simulink model "parrot_communication_host"  (R2022a)
settings: Solver=FixedStepAuto  StartTime=0.0  StopTime=50  FixedStep=0.05  RelTol=1e-3
undefined symbols (not defined in the file or in its folder): f
libraries: instrumentlib x2
settings Model: ExtModeTrigDuration=80  Creator=The MathWorks, Inc.  LastModifiedBy=The MathWorks, Inc.
settings SolverCC: AlgebraicLoopSolver=TrustRegion
settings DataIOCC: ReturnWorkspaceOutputs=off
settings OptimizationCC: DefaultParameterBehavior=Inlined  EnhancedBackFolding=on  PassReuseOutputArgsAs=Individual arguments  MaxStackSize=64  OptimizeBlockOrder=speed  DifferentSizesBufferReuse=on  OptimizationCustomize=off  EfficientTunableParamExpr=on
settings DebuggingCC: ParameterTunabilityLossMsg=error  UnconnectedInputMsg=warning  UnconnectedOutputMsg=warning  UnconnectedLineMsg=warning  SFMachineParentedDataDiag=warning  ArithmeticOperatorsInVariantConditions=warning
settings HardwareCC: ProdBitPerPointer=32  ProdBitPerSizeT=32  ProdBitPerPtrDiffT=32  ProdLargestAtomicInteger=Long  ProdWordSize=32  ProdHWDeviceType=ARM Compatible->ARM 9  UseEmbeddedCoderFeatures=off  UseSimulinkCoderFeatures=off
settings SFSimCC: SimUseLocalCustomCode=off  MATLABDynamicMemAlloc=off  CustomCodeUndefinedFunction=UseInterfaceOnly
settings RTWCC: SystemTargetFile=ert.tlc  TemplateMakefile=ert_default_tmf  GenerateReport=on  RTWUseLocalCustomCode=off  Toolchain=Sourcery G++ Lite GNU Toolchain for Drones  IncludeHyperlinkInReport=on  LaunchReport=on  GenerateTraceInfo=on  GenerateTraceReport=on  GenerateTraceReportSl=on  GenerateTraceReportSf=on  GenerateTraceReportEml=on
settings CodeAppCC: ForceParamTrailComments=on  IgnoreCustomStorageClasses=off  OperatorAnnotations=on  SimulinkDataObjDesc=on  SFDataObjDesc=on  InsertBlockDesc=on
settings ERTTargetCC: InlinedParameterPlacement=NonHierarchical  ERTCustomFileTemplate=example_file_process.tlc

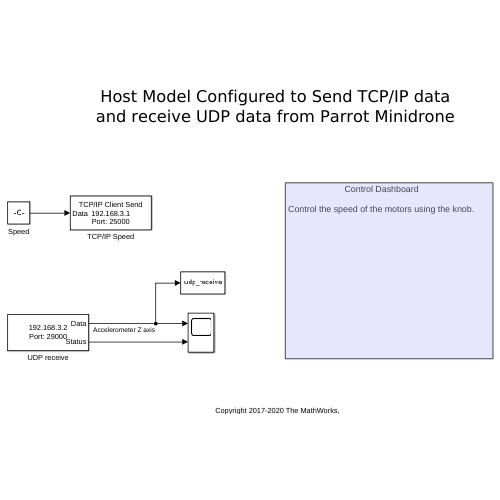
[thumbnail: Simulink's stored preview of the top-level diagram]
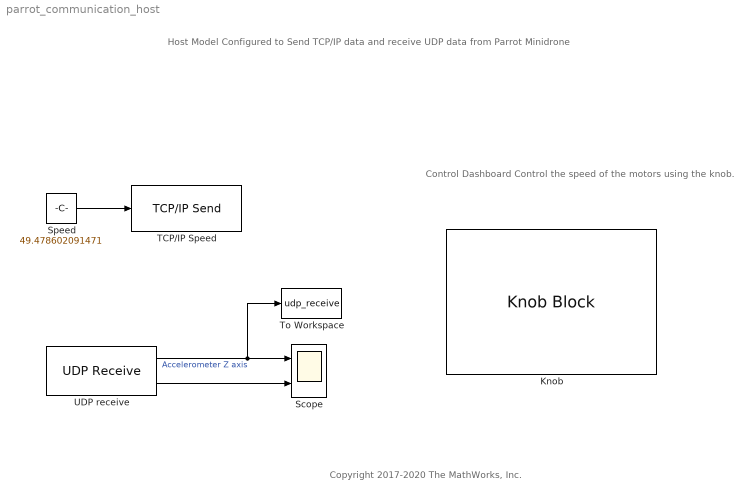
== system parrot_communication_host ==
  note: Control Dashboard
      |
      | Control the speed of the motors using the knob.
  note: Copyright 2017-2020 The MathWorks, Inc.
  note: Host Model Configured to Send TCP/IP data
      | and receive UDP data from Parrot Minidrone
  Knob : KnobBlock
  Scope : Scope  NumInputPorts=2
  "Speed " : Constant  Value=49.478602091471  SampleTime=0.05
  TCP/IP Speed : instrumentlib/TCP//IP Send  Host=192.168.3.1  Port=25000  ByteOrder=big-endian  EnableBlockingMode=off  Timeout=10  TransferDelay=off  SimulateUsing=Interpreted execution
  To Workspace : ToWorkspace  VariableName=udp_receive  SaveFormat=Timeseries  SampleTime=-1
  UDP receive : instrumentlib/UDP Receive  Host=192.168.3.5  Port=29000  LocalPort=29000  EnablePortSharing=off  GetLatestData=off  DataSize=1  DataType=single  ASCIIFormatting=%f,  Terminator=LF  ByteOrder=LittleEndian  EnableBlockingMode=off  Timeout=10  SampleTime=1  LocalAddress=192.168.3.2
  wires:
  "Speed "/1 -> TCP/IP Speed/1
  UDP receive/1 -> To Workspace/1, Scope/1  "Accelerometer Z axis"
  UDP receive/2 -> Scope/2
